simulink model "Copy_of_VTOLTiltrotor"  (R2024a)
settings: configuration reference "VTOLConfiguration" (kept outside this file)
undefined symbols (not defined in the file): airspeed, Battery, BCE12, BCE_Set_init, BMS_Controller_State, C, Cell10_P, Cell11_P, Cell12_P, Cell1_N, Cell1_P, Cell2_P, Cell3_P, Cell4_P, Cell5_P, Cell6_P, Cell7_P, Cell8_P, Cell9_P, Cell_Temperatures, Cell_Voltages, Charging_State, CityMission, control, controlParams, ControlSampleTime, CriticalTiltAngle, currentFactor, CV_Gain, ddx, ddy, ddz, Device_01, DiscIntNeverNeededParam, dx, dy, dz, Earth, env, F, F28379D_ADC_MaxCount, F28379D_ADC_Vmax, FixedWingMission, flightState, Foc_Ki_IxTcpu, Foc_Ki_S, Foc_Kp_I, Foc_Kp_S, fractalcoef, FSState, FWControlParams, HoverMission, I_cc, Ia_offset, Ib_offset, iniRoll, initPitch, iniYaw, IO334, IO334_DAC_Vmax ... (+55)
libraries: slrealtimeethercatlib x109, simulink x81, fl_lib x65, slpidlib x49, mcbcontrolslib x48, nesl_utility x43, speedgoatlib_hdlCoder_IO3xx x31, canmsglib x17, slrealtimeutilitieslib x13, mcbhdlplantlib x13, speedgoatlib_IO611 x12, dspstat3 x12
(part 3 of 20)

== system Copy_of_VTOLTiltrotor/Dynamics/Force and Moments ==
  note: Weather Model - Wind model is disabled by default. To enable wind model, run Wind = 0 and configure the wind model in the Weather Model subsystem.
      |
      | Aerodynamic Forces - Computes aerodynamic forces of the UAV. To modify the aerodynamic derivatives of the UAV, modify the uavParam.aero struct with your own data, or use the Aerodynamic Forces and Moments block from Aerospace Blockset
      |
      | Propulsion - Models the propulsion system. Open this subsystem to configure the rotor direction, tilt angle, etc.
  Actuator : Inport
  CtrlSurfaces : Inport  Port=2
  States : Inport  Port=3
  Add : Sum  Inputs=++++
  Add1 : Sum
  AeroSwitch : Constant  Value=0
  Aerodynamic Drag : Subsystem
  Aerodynamic Forces : Subsystem
  Bus Selector : BusSelector  OutputSignals=DCMbe,Vb
  Bus Selector3 : BusSelector  OutputSignals=Xe,Euler
  Constant4 : Constant  Value=0
  Constant5 : Constant  Value=0
  Gravity : Subsystem
  Propulsion : Subsystem
  Switch : Switch  Criteria=u2 > Threshold  SaturateOnIntegerOverflow=off  InputSameDT=off
  Switch1 : Switch  Criteria=u2 > Threshold  SaturateOnIntegerOverflow=off  InputSameDT=off
  Weather Model : Subsystem  Variant=on  VariantControl=Weather Model
  F : Outport
  M : Outport  Port=2
  RotorParams : Outport  Port=3
  AirData : Outport  Port=4
  wires:
  Bus Selector/1 -> Gravity/1(DCM_be), Aerodynamic Drag/1(DCM_be)  "<DCMbe>"
  Propulsion/3(F) -> Add/1
  Gravity/1(F_g) -> Add/2  "Gravity Force"
  Aerodynamic Drag/1(F_d) -> Add/4  "Drag Force"
  Bus Selector/2 -> Aerodynamic Drag/2(Vb)  "<Vb>"
  Add/1 -> F/1
  States/1 -> Bus Selector3/1, Bus Selector/1, Aerodynamic Forces/4(UAVState), Propulsion/2(States)  "States"
  CtrlSurfaces/1 -> Aerodynamic Forces/3(CtrlSurfaces)
  Add1/1 -> M/1
  Propulsion/2(M) -> Add1/2
  [AeroForce] -> Add/3  "Aerodynamic Force"
  Aerodynamic Forces/2(F) -> Switch/1
  Switch/1 -> [AeroForce]
  Constant4/1 -> Switch/3
  AeroSwitch/1 -> Switch/2, Switch1/2
  Constant5/1 -> Switch1/3
  Switch1/1 -> Add1/1, [AeroMoment]
  Aerodynamic Forces/3(M) -> Switch1/1
  Actuator/1 -> Propulsion/1(Actuator)
  Propulsion/1(RotorParameters) -> RotorParams/1
  Aerodynamic Forces/1(AirData) -> AirData/1, Weather Model/1(AirData)  "Air Data"
  Bus Selector3/1 -> Weather Model/2(Xe)  "<Xe>"
  Bus Selector3/2 -> Weather Model/3(Euler)  "<Euler>"
  Weather Model/1(Wind_e) -> Aerodynamic Forces/1(Wind_e)
  Weather Model/2(Rho) -> Aerodynamic Forces/2(Rho)

== system Copy_of_VTOLTiltrotor/Dynamics/Ground Truth Bus ==
  Ve : Inport
  Xe : Inport  Port=2
  Euler : Inport  Port=3
  DCMbe : Inport  Port=4
  Vb : Inport  Port=5
  pqr : Inport  Port=6
  Abb : Inport  Port=7
  Abe : Inport  Port=8
  RotorParams : Inport  Port=9
  AirData : Inport  Port=10
  Bus Creator : BusCreator  Inputs=13
  Bus Selector : BusSelector  OutputSignals=airspeed
  Direction Cosine Matrix to Quaternions : sharedtransform/Direction Cosine Matrix  to Quaternions  aMode=0  action=None  tolerance=eps(2)
      settings: LibrarySourceBlock=|
      | aerolibtransform2/Direction Cosine Matrix
      | to Quaternions
  MATLAB Function1 : MATLAB Function  TreatAsAtomicUnit=on
  Ground Truth : Outport
  wires:
  pqr/1 -> Bus Creator/6
  Xe/1 -> Bus Creator/2
  Bus Creator/1 -> Ground Truth/1
  DCMbe/1 -> Direction Cosine Matrix to Quaternions/1, Bus Creator/4
  Euler/1 -> Bus Creator/3
  Vb/1 -> Bus Creator/5
  Abb/1 -> Bus Creator/7
  AirData/1 -> Bus Selector/1
  Bus Selector/1 -> Bus Creator/9  "<airspeed>"
  Direction Cosine Matrix to Quaternions/1 -> Bus Creator/10  "q"
  RotorParams/1 -> Bus Creator/8  "RotorParameters"
  Abe/1 -> Bus Creator/11  "Abe"
  MATLAB Function1/2(gndSpeed) -> Bus Creator/13  "gndspeed"
  MATLAB Function1/1(course) -> Bus Creator/12  "course"
  Ve/1 -> MATLAB Function1/1(vxyz), Bus Creator/1

== system Copy_of_VTOLTiltrotor/Dynamics/Variant Subsystem ==
  UAVStates : Inport
  No Sensors : Subsystem  VariantControl=SensorType==0
  Sensors : Subsystem  VariantControl=SensorType==1
  SensorData : Outport

== system Copy_of_VTOLTiltrotor/Flight Controller/Autopilot ==
  note: To modify the output bus interfaces, run open("exampleHelperDefineDigitalTwinInterface.m")
  HoverCommands : Inport
  FixedWingSP : Inport  Port=2
  AAC : Inport  Port=3
  CtrlMode : Inport  Port=4
  FlightMode : Inport  Port=5
  EstimatedStates : Inport  Port=6
  Bus Selector : BusSelector  OutputSignals=inTransition
  Bus Selector1 : BusSelector  OutputSignals=TransitionCondition
  Bus Selector2 : BusSelector  OutputSignals=w1,w2,w3,w4
  Filter or Estimator : Subsystem
  Fixed Wing Controller : Subsystem  Variant=on  VariantControl=Fixed Wing Controller
  Manual Control : Subsystem
  Multicopter Controller : Subsystem
  Scheduler : Subsystem  SystemSampleTime=0.005
  Scope : Scope  NumInputPorts=4
  Tilt Scheduler : Subsystem
  MotorActuatorCommands : Outport
  CtrlSurfaceCmds : Outport  Port=2
  wires:
  EstimatedStates/1 -> Filter or Estimator/1(SensorData)
  Multicopter Controller/1(MixerCommands) -> Scheduler/1(MotorCommands)
  Tilt Scheduler/1(TiltAngle) -> Scheduler/2(TiltSchedule)
  Fixed Wing Controller/1(Actuator) -> Scheduler/6(FixedWingActuators)
  CtrlMode/1 -> Bus Selector1/1, Fixed Wing Controller/2(Control Mode), Bus Selector/1
  Manual Control/1(AERT) -> Fixed Wing Controller/5(AERT)
  Scheduler/1(MotorActuatorCommands) -> Bus Selector2/1, MotorActuatorCommands/1
  Scheduler/2(CtrlSurfaceCommands) -> CtrlSurfaceCmds/1
  HoverCommands/1 -> Multicopter Controller/1(Hover Commands)
  FlightMode/1 -> Tilt Scheduler/1(FlightMode)
  Filter or Estimator/1(States) -> Multicopter Controller/3(States), Fixed Wing Controller/1(States), Tilt Scheduler/2(States), Scheduler/4(States)
  AAC/1 -> Fixed Wing Controller/3(AAC SP)
  FixedWingSP/1 -> Fixed Wing Controller/4(FixedWingSP)
  [TransitionDone] -> Scheduler/5(TransitionDone)
  Tilt Scheduler/2(FlightState) -> Scheduler/3(FlightState)
  Bus Selector/1 -> Multicopter Controller/2(InTransition)  "<inTransition>"
  Bus Selector1/1 -> [TransitionDone]  "<TransitionCondition>"
  Bus Selector2/1 -> Scope/1  "<w1>"
  Bus Selector2/2 -> Scope/2  "<w2>"
  Bus Selector2/3 -> Scope/3  "<w3>"
  Bus Selector2/4 -> Scope/4  "<w4>"

== system Copy_of_VTOLTiltrotor/Flight Controller/Estimator ==
  SensorData : Inport
  Estimation Filter : Subsystem  VariantControl=SensorType==1
  Ground Truth : Subsystem  VariantControl=SensorType==0
  EstimatedStates : Outport

== system Copy_of_VTOLTiltrotor/Flight Controller/Ground Control Station ==
  note: Set mission type. In the project shortcut, choose between:
      | Hover mission by selecting Guidance Mode under Hover
      | Fixed wing mission by selecting Guidance Mode under Fixed wing
      | Transition mission by selecting Set Up Full Transition Mission under Transition
      | City mission by selecting Set Up City Mission under Photorealistic Simulation
  UAVState : Inport
  Get Flight Mission : Subsystem  Variant=on  VariantControlMode=label  LabelModeActiveChoice=useQGC==0
  Global Mission : Outport
  wires:
  Get Flight Mission/1("Mission ") -> Global Mission/1
  UAVState/1 -> Get Flight Mission/1(UAVState)

== system Copy_of_VTOLTiltrotor/Flight Controller/Guidance Test Bench ==
  note: Set control type. In the project shortcut, choose between:
      | 1. Manual control by selecting Manual Mode under Hover and open the subsystem to manually control the UAV in hover mode.
      | 2. Guidance testbench with prebuilt mission by selecting Guidance Mod e in the project shortcut.
  Aircraft States : Inport
  Global Mission : Inport  Port=2
  ControlType : Subsystem  Variant=on  VariantControl=Choice
  Rate Transition : RateTransition  OutPortSampleTime=0.005
  "Reference Tracking " : Subsystem
      settings: PortSchema="{\"entries\":[{\"content\":{\"sides\":[{\"content\":{\"connectorIds\":[\"In1\"]},\"type\":\"ConnectorPlacement.EquallySpacedRectSide\",\"uuid\":\"259d5f1e-a362-4dc0-8429-ef92dd781b31\"},{\"content\":{\"connectorIds\":[\"In2\",\"In3\"],\"side\":\"RIGHT\"},\"type\":\"ConnectorPlacement.EquallySpacedRectSide\",\"uuid\":\"8f699bfb-ab92-4bfa-94de-3c6c350a8a94\"},{\"content\":{\"connectorIds\":[],\"side\":\"TOP\"},\"type\":\"ConnectorPlacement.EquallySpacedRectSide\",\"uuid\":\"95dbffc6-e5b7-446a-adcb-afa0cff8c552\"}]},\"type\":\"ConnectorPlacement.EquallySpacedConnector\",\"uuid\":\"e657b5d9-4fa5-41f8-85e3-18a1074ff1cd\"}],\"packageUris\":[\"http://schema.mathworks.com/mf0/Connector/R2020b\"],\"version\":\"1.0\"}"
  HoverSP : Outport
  FixedWingSP : Outport  Port=2
  AACSP : Outport  Port=3
  ctrlMode : Outport  Port=4
  FlightMode : Outport  Port=5
  wires:
  Aircraft States/1 -> Rate Transition/1
  ControlType/1(HoverCmds) -> "Reference Tracking "/2(Position Command), HoverSP/1
  Global Mission/1 -> ControlType/2(Global Mission)
  ControlType/2(FixedWingSP) -> FixedWingSP/1
  ControlType/5(FlightMode) -> FlightMode/1
  ControlType/4(ctrlMode) -> ctrlMode/1
  ControlType/3(AACSP) -> "Reference Tracking "/3(AAC Commands), AACSP/1
  Rate Transition/1 -> "Reference Tracking "/1(State), ControlType/1(Aircraft States)

== system Copy_of_VTOLTiltrotor/Motor Control/Actuator To PWM for all motors ==
  Motor Commands : Inport
  Bus Creator : BusCreator  Inputs=6  OutDataTypeStr=Bus: RotorCntrlBus
  Bus Selector : BusSelector  OutputSignals=w1,w2,w3,w4,Tilt1,Tilt2
  Gain{,1..2,4} (4 alike) : Gain  Gain=1/(uavParam.motor.RPMMAX/60)
  Gain3 : Gain  Gain=1/(pi/2)
  Gain5 : Gain  Gain=1/(pi/2)
  To PWM : Outport
  wires:
  Motor Commands/1 -> Bus Selector/1
  Bus Selector/1 -> Gain/1  "<w1>"
  Bus Selector/3 -> Gain1/1  "<w3>"
  Bus Selector/2 -> Gain4/1  "<w2>"
  Bus Selector/4 -> Gain2/1  "<w4>"
  Bus Selector/5 -> Gain3/1  "<Tilt1>"
  Bus Selector/6 -> Gain5/1  "<Tilt2>"
  Gain/1 -> Bus Creator/1  "w1"
  Gain4/1 -> Bus Creator/2  "w2"
  Gain1/1 -> Bus Creator/3  "w3"
  Gain2/1 -> Bus Creator/4  "w4"
  Gain3/1 -> Bus Creator/5  "Tilt1"
  Gain5/1 -> Bus Creator/6  "Tilt2"
  Bus Creator/1 -> To PWM/1

== system Copy_of_VTOLTiltrotor/Motor Control/Actuator To RPM for 1 motor ==
  Motor Commands : Inport
  Gain : Gain  Gain=10
  Selector : Selector  InputPortWidth=6  IndexOptions=Index vector (dialog)  Indices=[1]  OutputSizes=1
  RPM : Outport
  wires:
  Motor Commands/1 -> Selector/1
  Selector/1 -> Gain/1
  Gain/1 -> RPM/1

== system Copy_of_VTOLTiltrotor/Motor Control/Actuator To RPM for 1 motor1 ==
  Motor Commands : Inport
  Gain : Gain  Gain=10
  Selector : Selector  InputPortWidth=6  IndexOptions=Index vector (dialog)  Indices=[2]  OutputSizes=1
  RPM : Outport
  wires:
  Motor Commands/1 -> Selector/1
  Selector/1 -> Gain/1
  Gain/1 -> RPM/1

== system Copy_of_VTOLTiltrotor/Motor Control/Actuator To RPM for 1 motor2 ==
  Motor Commands : Inport
  Gain : Gain  Gain=10
  Selector : Selector  InputPortWidth=6  IndexOptions=Index vector (dialog)  Indices=[3]  OutputSizes=1
  RPM : Outport
  wires:
  Motor Commands/1 -> Selector/1
  Selector/1 -> Gain/1
  Gain/1 -> RPM/1

== system Copy_of_VTOLTiltrotor/Motor Control/Actuator To RPM for 1 motor3 ==
  Motor Commands : Inport
  Gain : Gain  Gain=10
  Selector : Selector  InputPortWidth=6  IndexOptions=Index vector (dialog)  Indices=[4]  OutputSizes=1
  RPM : Outport
  wires:
  Motor Commands/1 -> Selector/1
  Selector/1 -> Gain/1
  Gain/1 -> RPM/1

== system Copy_of_VTOLTiltrotor/Motor Control/Controller ==
  Iab : Inport
  QAE_MIL_fbk : Inport  Port=2
  EnablePWM : Inport  Port=3
  Closed_Loop_FOC : Inport  Port=4
  Speed_CMD_RPM : Inport  Port=5
  Controller_Parameters : Inport  Port=6
  Controller_HIL_CAN : Subsystem  VariantControl=strcmp(get_param(['VTOLTiltrotor/Motor Control/SimulationVariant'], 'Value'),'3')
  Controller_MIL : Subsystem  VariantControl=(default)
  Controller_fbk : Outport
  Simu_config : Outport  Port=2

== system Copy_of_VTOLTiltrotor/Motor Control/Controller Parameters ==
  Controller_Parameters : BusCreator  Inputs=6
  Controller_Parameters1 : BusCreator  Inputs=6
  Default Values : Constant  OutDataTypeStr=boolean  SampleTime=Ts_UI
  Foc_Ki_S : Constant  Value=Foc_Ki_S  OutDataTypeStr=single
  Foc_Kp_I : Constant  Value=Foc_Kp_I  OutDataTypeStr=single
  Foc_Kp_S : Constant  Value=Foc_Kp_S  OutDataTypeStr=single
  Ia Offset : Constant  Value=Ia_offset  OutDataTypeStr=single
  Ia_offset : Constant  Value=Ia_offset  OutDataTypeStr=single  SampleTime=Ts_UI
  Ib Offset : Constant  Value=Ib_offset  OutDataTypeStr=single
  Ib_offset : Constant  Value=Ib_offset  OutDataTypeStr=single  SampleTime=Ts_UI
  Ki_S : Constant  Value=0.1  OutDataTypeStr=single  SampleTime=Ts_UI
  Ki_i*Tcpu : Constant  Value=Foc_Ki_IxTcpu  OutDataTypeStr=single  SampleTime=Ts_UI
  Ki_i*Tcpu1 : Constant  Value=Foc_Ki_IxTcpu  OutDataTypeStr=single
  Kp_I : Constant  Value=Foc_Kp_I  OutDataTypeStr=single  SampleTime=Ts_UI
  Kp_S : Constant  Value=0.1  OutDataTypeStr=single  SampleTime=Ts_UI
  Rate Transition : RateTransition  OutPortSampleTime=Ts_UI
  Switch : Switch  Criteria=u2 ~= 0  SaturateOnIntegerOverflow=off  InputSameDT=off
  Controller Parameters : Outport
  wires:
  Ia_offset/1 -> Controller_Parameters/5  "Ia_offset"
  Foc_Kp_S/1 -> Controller_Parameters1/1  "Kp_S"
  Ia Offset/1 -> Controller_Parameters1/5  "Ia_offset"
  Ib Offset/1 -> Controller_Parameters1/6  "Ib_offset"
  Controller_Parameters/1 -> Switch/3
  Foc_Ki_S/1 -> Controller_Parameters1/2  "Ki_S"
  Foc_Kp_I/1 -> Controller_Parameters1/3  "Kp_I"
  Controller_Parameters1/1 -> Rate Transition/1
  Ib_offset/1 -> Controller_Parameters/6  "Ib_offset"
  Ki_i*Tcpu/1 -> Controller_Parameters/4  "Ki_IxTcpu"
  Ki_S/1 -> Controller_Parameters/2  "Ki_S"
  Ki_i*Tcpu1/1 -> Controller_Parameters1/4  "Ki_IxTcpu"
  Kp_I/1 -> Controller_Parameters/3  "Kp_I"
  Kp_S/1 -> Controller_Parameters/1  "Kp_S"
  Switch/1 -> Controller Parameters/1
  Rate Transition/1 -> Switch/1
  Default Values/1 -> Switch/2  "Default Values"

== system Copy_of_VTOLTiltrotor/Motor Control/Controller Parameters1 ==
  Controller_Parameters : BusCreator  Inputs=6
  Controller_Parameters1 : BusCreator  Inputs=6
  Default Values : Constant  OutDataTypeStr=boolean  SampleTime=Ts_UI
  Foc_Ki_S : Constant  Value=Foc_Ki_S  OutDataTypeStr=single
  Foc_Kp_I : Constant  Value=Foc_Kp_I  OutDataTypeStr=single
  Foc_Kp_S : Constant  Value=Foc_Kp_S  OutDataTypeStr=single
  Ia Offset : Constant  Value=Ia_offset  OutDataTypeStr=single
  Ia_offset : Constant  Value=Ia_offset  OutDataTypeStr=single  SampleTime=Ts_UI
  Ib Offset : Constant  Value=Ib_offset  OutDataTypeStr=single
  Ib_offset : Constant  Value=Ib_offset  OutDataTypeStr=single  SampleTime=Ts_UI
  Ki_S : Constant  Value=0.1  OutDataTypeStr=single  SampleTime=Ts_UI
  Ki_i*Tcpu : Constant  Value=Foc_Ki_IxTcpu  OutDataTypeStr=single  SampleTime=Ts_UI
  Ki_i*Tcpu1 : Constant  Value=Foc_Ki_IxTcpu  OutDataTypeStr=single
  Kp_I : Constant  Value=Foc_Kp_I  OutDataTypeStr=single  SampleTime=Ts_UI
  Kp_S : Constant  Value=0.1  OutDataTypeStr=single  SampleTime=Ts_UI
  Rate Transition : RateTransition  OutPortSampleTime=Ts_UI
  Switch : Switch  Criteria=u2 ~= 0  SaturateOnIntegerOverflow=off  InputSameDT=off
  Controller Parameters : Outport
  wires:
  Ia_offset/1 -> Controller_Parameters/5  "Ia_offset"
  Foc_Kp_S/1 -> Controller_Parameters1/1  "Kp_S"
  Ia Offset/1 -> Controller_Parameters1/5  "Ia_offset"
  Ib Offset/1 -> Controller_Parameters1/6  "Ib_offset"
  Controller_Parameters/1 -> Switch/3
  Foc_Ki_S/1 -> Controller_Parameters1/2  "Ki_S"
  Foc_Kp_I/1 -> Controller_Parameters1/3  "Kp_I"
  Controller_Parameters1/1 -> Rate Transition/1
  Ib_offset/1 -> Controller_Parameters/6  "Ib_offset"
  Ki_i*Tcpu/1 -> Controller_Parameters/4  "Ki_IxTcpu"
  Ki_S/1 -> Controller_Parameters/2  "Ki_S"
  Ki_i*Tcpu1/1 -> Controller_Parameters1/4  "Ki_IxTcpu"
  Kp_I/1 -> Controller_Parameters/3  "Kp_I"
  Kp_S/1 -> Controller_Parameters/1  "Kp_S"
  Switch/1 -> Controller Parameters/1
  Rate Transition/1 -> Switch/1
  Default Values/1 -> Switch/2  "Default Values"

== system Copy_of_VTOLTiltrotor/Motor Control/Controller Parameters2 ==
  Controller_Parameters : BusCreator  Inputs=6
  Controller_Parameters1 : BusCreator  Inputs=6
  Default Values : Constant  OutDataTypeStr=boolean  SampleTime=Ts_UI
  Foc_Ki_S : Constant  Value=Foc_Ki_S  OutDataTypeStr=single
  Foc_Kp_I : Constant  Value=Foc_Kp_I  OutDataTypeStr=single
  Foc_Kp_S : Constant  Value=Foc_Kp_S  OutDataTypeStr=single
  Ia Offset : Constant  Value=Ia_offset  OutDataTypeStr=single
  Ia_offset : Constant  Value=Ia_offset  OutDataTypeStr=single  SampleTime=Ts_UI
  Ib Offset : Constant  Value=Ib_offset  OutDataTypeStr=single
  Ib_offset : Constant  Value=Ib_offset  OutDataTypeStr=single  SampleTime=Ts_UI
  Ki_S : Constant  Value=0.1  OutDataTypeStr=single  SampleTime=Ts_UI
  Ki_i*Tcpu : Constant  Value=Foc_Ki_IxTcpu  OutDataTypeStr=single  SampleTime=Ts_UI
  Ki_i*Tcpu1 : Constant  Value=Foc_Ki_IxTcpu  OutDataTypeStr=single
  Kp_I : Constant  Value=Foc_Kp_I  OutDataTypeStr=single  SampleTime=Ts_UI
  Kp_S : Constant  Value=0.1  OutDataTypeStr=single  SampleTime=Ts_UI
  Rate Transition : RateTransition  OutPortSampleTime=Ts_UI
  Switch : Switch  Criteria=u2 ~= 0  SaturateOnIntegerOverflow=off  InputSameDT=off
  Controller Parameters : Outport
  wires:
  Ia_offset/1 -> Controller_Parameters/5  "Ia_offset"
  Foc_Kp_S/1 -> Controller_Parameters1/1  "Kp_S"
  Ia Offset/1 -> Controller_Parameters1/5  "Ia_offset"
  Ib Offset/1 -> Controller_Parameters1/6  "Ib_offset"
  Controller_Parameters/1 -> Switch/3
  Foc_Ki_S/1 -> Controller_Parameters1/2  "Ki_S"
  Foc_Kp_I/1 -> Controller_Parameters1/3  "Kp_I"
  Controller_Parameters1/1 -> Rate Transition/1
  Ib_offset/1 -> Controller_Parameters/6  "Ib_offset"
  Ki_i*Tcpu/1 -> Controller_Parameters/4  "Ki_IxTcpu"
  Ki_S/1 -> Controller_Parameters/2  "Ki_S"
  Ki_i*Tcpu1/1 -> Controller_Parameters1/4  "Ki_IxTcpu"
  Kp_I/1 -> Controller_Parameters/3  "Kp_I"
  Kp_S/1 -> Controller_Parameters/1  "Kp_S"
  Switch/1 -> Controller Parameters/1
  Rate Transition/1 -> Switch/1
  Default Values/1 -> Switch/2  "Default Values"

== system Copy_of_VTOLTiltrotor/Motor Control/Controller Parameters3 ==
  Controller_Parameters : BusCreator  Inputs=6
  Controller_Parameters1 : BusCreator  Inputs=6
  Default Values : Constant  OutDataTypeStr=boolean  SampleTime=Ts_UI
  Foc_Ki_S : Constant  Value=Foc_Ki_S  OutDataTypeStr=single
  Foc_Kp_I : Constant  Value=Foc_Kp_I  OutDataTypeStr=single
  Foc_Kp_S : Constant  Value=Foc_Kp_S  OutDataTypeStr=single
  Ia Offset : Constant  Value=Ia_offset  OutDataTypeStr=single
  Ia_offset : Constant  Value=Ia_offset  OutDataTypeStr=single  SampleTime=Ts_UI
  Ib Offset : Constant  Value=Ib_offset  OutDataTypeStr=single
  Ib_offset : Constant  Value=Ib_offset  OutDataTypeStr=single  SampleTime=Ts_UI
  Ki_S : Constant  Value=0.1  OutDataTypeStr=single  SampleTime=Ts_UI
  Ki_i*Tcpu : Constant  Value=Foc_Ki_IxTcpu  OutDataTypeStr=single  SampleTime=Ts_UI
  Ki_i*Tcpu1 : Constant  Value=Foc_Ki_IxTcpu  OutDataTypeStr=single
  Kp_I : Constant  Value=Foc_Kp_I  OutDataTypeStr=single  SampleTime=Ts_UI
  Kp_S : Constant  Value=0.1  OutDataTypeStr=single  SampleTime=Ts_UI
  Rate Transition : RateTransition  OutPortSampleTime=Ts_UI
  Switch : Switch  Criteria=u2 ~= 0  SaturateOnIntegerOverflow=off  InputSameDT=off
  Controller Parameters : Outport
  wires:
  Ia_offset/1 -> Controller_Parameters/5  "Ia_offset"
  Foc_Kp_S/1 -> Controller_Parameters1/1  "Kp_S"
  Ia Offset/1 -> Controller_Parameters1/5  "Ia_offset"
  Ib Offset/1 -> Controller_Parameters1/6  "Ib_offset"
  Controller_Parameters/1 -> Switch/3
  Foc_Ki_S/1 -> Controller_Parameters1/2  "Ki_S"
  Foc_Kp_I/1 -> Controller_Parameters1/3  "Kp_I"
  Controller_Parameters1/1 -> Rate Transition/1
  Ib_offset/1 -> Controller_Parameters/6  "Ib_offset"
  Ki_i*Tcpu/1 -> Controller_Parameters/4  "Ki_IxTcpu"
  Ki_S/1 -> Controller_Parameters/2  "Ki_S"
  Ki_i*Tcpu1/1 -> Controller_Parameters1/4  "Ki_IxTcpu"
  Kp_I/1 -> Controller_Parameters/3  "Kp_I"
  Kp_S/1 -> Controller_Parameters/1  "Kp_S"
  Switch/1 -> Controller Parameters/1
  Rate Transition/1 -> Switch/1
  Default Values/1 -> Switch/2  "Default Values"

== system Copy_of_VTOLTiltrotor/Motor Control/Controller1 ==
  Iab : Inport
  QAE_MIL_fbk : Inport  Port=2
  EnablePWM : Inport  Port=3
  Closed_Loop_FOC : Inport  Port=4
  Speed_CMD_RPM : Inport  Port=5
  Controller_Parameters : Inport  Port=6
  Controller_MIL : Subsystem  VariantControl=(default)
  Controller_fbk : Outport
  Simu_config : Outport  Port=2

== system Copy_of_VTOLTiltrotor/Motor Control/Controller2 ==
  Iab : Inport
  QAE_MIL_fbk : Inport  Port=2
  EnablePWM : Inport  Port=3
  Closed_Loop_FOC : Inport  Port=4
  Speed_CMD_RPM : Inport  Port=5
  Controller_Parameters : Inport  Port=6
  Controller_MIL : Subsystem  VariantControl=(default)
  Controller_fbk : Outport
  Simu_config : Outport  Port=2

== system Copy_of_VTOLTiltrotor/Motor Control/Controller3 ==
  Iab : Inport
  QAE_MIL_fbk : Inport  Port=2
  EnablePWM : Inport  Port=3
  Closed_Loop_FOC : Inport  Port=4
  Speed_CMD_RPM : Inport  Port=5
  Controller_Parameters : Inport  Port=6
  Controller_MIL : Subsystem  VariantControl=(default)
  Controller_fbk : Outport
  Simu_config : Outport  Port=2

== system Copy_of_VTOLTiltrotor/Motor Control/Controller_fbk_signals ==
  Controller_fbk : Inport
  Data Type Conversion : DataTypeConversion  OutDataTypeStr=boolean  SaturateOnIntegerOverflow=off  RndMeth=Floor
  Demux : Demux
  Terminator{,1..3} (4 alike) : Terminator
  wires:
  Demux/1 -> Terminator1/1  "Speed_fbk"
  Controller_fbk/1 -> Demux/1
  Demux/2 -> Terminator3/1  "Encoder_Pos_fbk"
  Demux/4 -> Data Type Conversion/1  "Spd_Pot_fdk"
  Demux/3 -> Terminator2/1  "Speed_Cmd_fbk"
  Data Type Conversion/1 -> Terminator/1  "Spd_pot_enable"

== system Copy_of_VTOLTiltrotor/Motor Control/Controller_fbk_signals1 ==
  Controller_fbk : Inport
  Data Type Conversion : DataTypeConversion  OutDataTypeStr=boolean  SaturateOnIntegerOverflow=off  RndMeth=Floor
  Demux : Demux
  Terminator{,1..3} (4 alike) : Terminator
  wires:
  Demux/1 -> Terminator1/1  "Speed_fbk"
  Controller_fbk/1 -> Demux/1
  Demux/2 -> Terminator3/1  "Encoder_Pos_fbk"
  Demux/4 -> Data Type Conversion/1  "Spd_Pot_fdk"
  Demux/3 -> Terminator2/1  "Speed_Cmd_fbk"
  Data Type Conversion/1 -> Terminator/1  "Spd_pot_enable"

== system Copy_of_VTOLTiltrotor/Motor Control/Controller_fbk_signals2 ==
  Controller_fbk : Inport
  Data Type Conversion : DataTypeConversion  OutDataTypeStr=boolean  SaturateOnIntegerOverflow=off  RndMeth=Floor
  Demux : Demux
  Terminator{,1..3} (4 alike) : Terminator
  wires:
  Demux/1 -> Terminator1/1  "Speed_fbk"
  Controller_fbk/1 -> Demux/1
  Demux/2 -> Terminator3/1  "Encoder_Pos_fbk"
  Demux/4 -> Data Type Conversion/1  "Spd_Pot_fdk"
  Demux/3 -> Terminator2/1  "Speed_Cmd_fbk"
  Data Type Conversion/1 -> Terminator/1  "Spd_pot_enable"

== system Copy_of_VTOLTiltrotor/Motor Control/Controller_fbk_signals3 ==
  Controller_fbk : Inport
  Data Type Conversion : DataTypeConversion  OutDataTypeStr=boolean  SaturateOnIntegerOverflow=off  RndMeth=Floor
  Demux : Demux
  Terminator{,1..3} (4 alike) : Terminator
  wires:
  Demux/1 -> Terminator1/1  "Speed_fbk"
  Controller_fbk/1 -> Demux/1
  Demux/2 -> Terminator3/1  "Encoder_Pos_fbk"
  Demux/4 -> Data Type Conversion/1  "Spd_Pot_fdk"
  Demux/3 -> Terminator2/1  "Speed_Cmd_fbk"
  Data Type Conversion/1 -> Terminator/1  "Spd_pot_enable"

== system Copy_of_VTOLTiltrotor/Motor Control/Fault Trigering ==
  AND : Logic  Inputs=3  IconShape=distinctive  AllPortsSameDT=off  OutDataTypeStr=boolean
  Bit to Integer Converter : simulink/Logic and Bit Operations/Bit to Integer Converter  nbits=32  bitOrder=LSB first  signedOutputValues=Unsigned  outDtype=uint32  outDtypeSigned=Inherit via internal rule
  Close_An : Constant  Value=0  OutDataTypeStr=boolean  SampleTime=Ts_UI
  Close_Ap : Constant  Value=0  OutDataTypeStr=boolean  SampleTime=Ts_UI
  Close_Bn : Constant  Value=0  OutDataTypeStr=boolean  SampleTime=Ts_UI
  Close_Bp : Constant  Value=0  OutDataTypeStr=boolean  SampleTime=Ts_UI
  Close_Cn : Constant  Value=0  OutDataTypeStr=boolean  SampleTime=Ts_UI
  Close_Cp : Constant  Value=0  OutDataTypeStr=boolean  SampleTime=Ts_UI
  Constant1 : Constant  Value=0  OutDataTypeStr=uint32
  Constant{14..15,20..25,32..36} (13 alike) : Constant  Value=0  OutDataTypeStr=boolean  SampleTime=Ts_UI
  Constant2 : Constant  OutDataTypeStr=boolean  SampleTime=Ts_UI
  Enable_Fault_UI : Constant  OutDataTypeStr=boolean  SampleTime=Ts_UI
  OR : Logic  Operator=OR  Inputs=18  IconShape=distinctive  AllPortsSameDT=off  OutDataTypeStr=boolean
  Open_An : Constant  Value=0  OutDataTypeStr=boolean  SampleTime=Ts_UI
  Open_Ap : Constant  Value=0  OutDataTypeStr=boolean  SampleTime=Ts_UI
  Open_Bn : Constant  Value=0  OutDataTypeStr=boolean  SampleTime=Ts_UI
  Open_Bp : Constant  Value=0  OutDataTypeStr=boolean  SampleTime=Ts_UI
  Open_Cn : Constant  Value=0  OutDataTypeStr=boolean  SampleTime=Ts_UI
  Open_Cp : Constant  Value=0  OutDataTypeStr=boolean  SampleTime=Ts_UI
  Short_A : Constant  Value=0  OutDataTypeStr=boolean  SampleTime=Ts_UI
  Short_AB : Constant  Value=0  OutDataTypeStr=boolean  SampleTime=Ts_UI
  Short_B : Constant  Value=0  OutDataTypeStr=boolean  SampleTime=Ts_UI
  Short_BC : Constant  Value=0  OutDataTypeStr=boolean  SampleTime=Ts_UI
  Short_C : Constant  Value=0  OutDataTypeStr=boolean  SampleTime=Ts_UI
  Short_CA : Constant  Value=0  OutDataTypeStr=boolean  SampleTime=Ts_UI
  Switch : Switch  Criteria=u2 > Threshold  SaturateOnIntegerOverflow=off  InputSameDT=off
  Terminator : Terminator
  Vector Concatenate : Concatenate  NumInputs=32
  Faults : Outport
  wires:
  Open_Cn/1 -> OR/12, Vector Concatenate/12
  Open_Cp/1 -> OR/9, Vector Concatenate/9
  Short_A/1 -> OR/1, Vector Concatenate/1
  Open_Bp/1 -> OR/8, Vector Concatenate/8
  Short_B/1 -> Vector Concatenate/2, OR/2
  Short_C/1 -> Vector Concatenate/3, OR/3
  Short_AB/1 -> Vector Concatenate/4, OR/4
  Short_BC/1 -> Vector Concatenate/5, OR/5
  Short_CA/1 -> OR/6, Vector Concatenate/6
  Constant36/1 -> Vector Concatenate/31
  Open_Bn/1 -> OR/11, Vector Concatenate/11
  Open_An/1 -> OR/10, Vector Concatenate/10
  Open_Ap/1 -> OR/7, Vector Concatenate/7
  Close_An/1 -> OR/16, Vector Concatenate/16
  Close_Ap/1 -> OR/13, Vector Concatenate/13
  Close_Cn/1 -> OR/18, Vector Concatenate/18
  Close_Bn/1 -> OR/17, Vector Concatenate/17
  Close_Cp/1 -> OR/15, Vector Concatenate/15
  Close_Bp/1 -> OR/14, Vector Concatenate/14
  Constant15/1 -> Vector Concatenate/24
  Constant14/1 -> Vector Concatenate/23
  Constant21/1 -> Vector Concatenate/20
  Constant20/1 -> Vector Concatenate/19
  Constant25/1 -> Vector Concatenate/26
  Constant24/1 -> Vector Concatenate/25
  Constant23/1 -> Vector Concatenate/22
  Constant22/1 -> Vector Concatenate/21
  Constant35/1 -> Vector Concatenate/30
  Constant34/1 -> Vector Concatenate/29
  Constant33/1 -> Vector Concatenate/28
  Constant32/1 -> Vector Concatenate/27
  Enable_Fault_UI/1 -> AND/3, Switch/2
  Vector Concatenate/1 -> Bit to Integer Converter/1
  Switch/1 -> Faults/1
  Bit to Integer Converter/1 -> Switch/1
  Constant1/1 -> Switch/3
  OR/1 -> AND/1
  AND/1 -> Terminator/1  "Fault_Present"
  Constant2/1 -> AND/2, Vector Concatenate/32

== system Copy_of_VTOLTiltrotor/Motor Control/Fault Trigering1 ==
  AND : Logic  Inputs=3  IconShape=distinctive  AllPortsSameDT=off  OutDataTypeStr=boolean
  Bit to Integer Converter : simulink/Logic and Bit Operations/Bit to Integer Converter  nbits=32  bitOrder=LSB first  signedOutputValues=Unsigned  outDtype=uint32  outDtypeSigned=Inherit via internal rule
  Close_An : Constant  Value=0  OutDataTypeStr=boolean  SampleTime=Ts_UI
  Close_Ap : Constant  Value=0  OutDataTypeStr=boolean  SampleTime=Ts_UI
  Close_Bn : Constant  Value=0  OutDataTypeStr=boolean  SampleTime=Ts_UI
  Close_Bp : Constant  Value=0  OutDataTypeStr=boolean  SampleTime=Ts_UI
  Close_Cn : Constant  Value=0  OutDataTypeStr=boolean  SampleTime=Ts_UI
  Close_Cp : Constant  Value=0  OutDataTypeStr=boolean  SampleTime=Ts_UI
  Constant1 : Constant  Value=0  OutDataTypeStr=uint32
  Constant{14..15,20..25,32..36} (13 alike) : Constant  Value=0  OutDataTypeStr=boolean  SampleTime=Ts_UI
  Constant2 : Constant  OutDataTypeStr=boolean  SampleTime=Ts_UI
  Enable_Fault_UI : Constant  OutDataTypeStr=boolean  SampleTime=Ts_UI
  OR : Logic  Operator=OR  Inputs=18  IconShape=distinctive  AllPortsSameDT=off  OutDataTypeStr=boolean
  Open_An : Constant  Value=0  OutDataTypeStr=boolean  SampleTime=Ts_UI
  Open_Ap : Constant  Value=0  OutDataTypeStr=boolean  SampleTime=Ts_UI
  Open_Bn : Constant  Value=0  OutDataTypeStr=boolean  SampleTime=Ts_UI
  Open_Bp : Constant  Value=0  OutDataTypeStr=boolean  SampleTime=Ts_UI
  Open_Cn : Constant  Value=0  OutDataTypeStr=boolean  SampleTime=Ts_UI
  Open_Cp : Constant  Value=0  OutDataTypeStr=boolean  SampleTime=Ts_UI
  Short_A : Constant  Value=0  OutDataTypeStr=boolean  SampleTime=Ts_UI
  Short_AB : Constant  Value=0  OutDataTypeStr=boolean  SampleTime=Ts_UI
  Short_B : Constant  Value=0  OutDataTypeStr=boolean  SampleTime=Ts_UI
  Short_BC : Constant  Value=0  OutDataTypeStr=boolean  SampleTime=Ts_UI
  Short_C : Constant  Value=0  OutDataTypeStr=boolean  SampleTime=Ts_UI
  Short_CA : Constant  Value=0  OutDataTypeStr=boolean  SampleTime=Ts_UI
  Switch : Switch  Criteria=u2 > Threshold  SaturateOnIntegerOverflow=off  InputSameDT=off
  Terminator : Terminator
  Vector Concatenate : Concatenate  NumInputs=32
  Faults : Outport
  wires:
  Open_Cn/1 -> OR/12, Vector Concatenate/12
  Open_Cp/1 -> OR/9, Vector Concatenate/9
  Short_A/1 -> OR/1, Vector Concatenate/1
  Open_Bp/1 -> OR/8, Vector Concatenate/8
  Short_B/1 -> Vector Concatenate/2, OR/2
  Short_C/1 -> Vector Concatenate/3, OR/3
  Short_AB/1 -> Vector Concatenate/4, OR/4
  Short_BC/1 -> Vector Concatenate/5, OR/5
  Short_CA/1 -> OR/6, Vector Concatenate/6
  Constant36/1 -> Vector Concatenate/31
  Open_Bn/1 -> OR/11, Vector Concatenate/11
  Open_An/1 -> OR/10, Vector Concatenate/10
  Open_Ap/1 -> OR/7, Vector Concatenate/7
  Close_An/1 -> OR/16, Vector Concatenate/16
  Close_Ap/1 -> OR/13, Vector Concatenate/13
  Close_Cn/1 -> OR/18, Vector Concatenate/18
  Close_Bn/1 -> OR/17, Vector Concatenate/17
  Close_Cp/1 -> OR/15, Vector Concatenate/15
  Close_Bp/1 -> OR/14, Vector Concatenate/14
  Constant15/1 -> Vector Concatenate/24
  Constant14/1 -> Vector Concatenate/23
  Constant21/1 -> Vector Concatenate/20
  Constant20/1 -> Vector Concatenate/19
  Constant25/1 -> Vector Concatenate/26
  Constant24/1 -> Vector Concatenate/25
  Constant23/1 -> Vector Concatenate/22
  Constant22/1 -> Vector Concatenate/21
  Constant35/1 -> Vector Concatenate/30
  Constant34/1 -> Vector Concatenate/29
  Constant33/1 -> Vector Concatenate/28
  Constant32/1 -> Vector Concatenate/27
  Enable_Fault_UI/1 -> AND/3, Switch/2
  Vector Concatenate/1 -> Bit to Integer Converter/1
  Switch/1 -> Faults/1
  Bit to Integer Converter/1 -> Switch/1
  Constant1/1 -> Switch/3
  OR/1 -> AND/1
  AND/1 -> Terminator/1  "Fault_Present"
  Constant2/1 -> AND/2, Vector Concatenate/32

== system Copy_of_VTOLTiltrotor/Motor Control/Fault Trigering2 ==
  AND : Logic  Inputs=3  IconShape=distinctive  AllPortsSameDT=off  OutDataTypeStr=boolean
  Bit to Integer Converter : simulink/Logic and Bit Operations/Bit to Integer Converter  nbits=32  bitOrder=LSB first  signedOutputValues=Unsigned  outDtype=uint32  outDtypeSigned=Inherit via internal rule
  Close_An : Constant  Value=0  OutDataTypeStr=boolean  SampleTime=Ts_UI
  Close_Ap : Constant  Value=0  OutDataTypeStr=boolean  SampleTime=Ts_UI
  Close_Bn : Constant  Value=0  OutDataTypeStr=boolean  SampleTime=Ts_UI
  Close_Bp : Constant  Value=0  OutDataTypeStr=boolean  SampleTime=Ts_UI
  Close_Cn : Constant  Value=0  OutDataTypeStr=boolean  SampleTime=Ts_UI
  Close_Cp : Constant  Value=0  OutDataTypeStr=boolean  SampleTime=Ts_UI
  Constant1 : Constant  Value=0  OutDataTypeStr=uint32
  Constant{14..15,20..25,32..36} (13 alike) : Constant  Value=0  OutDataTypeStr=boolean  SampleTime=Ts_UI
  Constant2 : Constant  OutDataTypeStr=boolean  SampleTime=Ts_UI
  Enable_Fault_UI : Constant  OutDataTypeStr=boolean  SampleTime=Ts_UI
  OR : Logic  Operator=OR  Inputs=18  IconShape=distinctive  AllPortsSameDT=off  OutDataTypeStr=boolean
  Open_An : Constant  Value=0  OutDataTypeStr=boolean  SampleTime=Ts_UI
  Open_Ap : Constant  Value=0  OutDataTypeStr=boolean  SampleTime=Ts_UI
  Open_Bn : Constant  Value=0  OutDataTypeStr=boolean  SampleTime=Ts_UI
  Open_Bp : Constant  Value=0  OutDataTypeStr=boolean  SampleTime=Ts_UI
  Open_Cn : Constant  Value=0  OutDataTypeStr=boolean  SampleTime=Ts_UI
  Open_Cp : Constant  Value=0  OutDataTypeStr=boolean  SampleTime=Ts_UI
  Short_A : Constant  Value=0  OutDataTypeStr=boolean  SampleTime=Ts_UI
  Short_AB : Constant  Value=0  OutDataTypeStr=boolean  SampleTime=Ts_UI
  Short_B : Constant  Value=0  OutDataTypeStr=boolean  SampleTime=Ts_UI
  Short_BC : Constant  Value=0  OutDataTypeStr=boolean  SampleTime=Ts_UI
  Short_C : Constant  Value=0  OutDataTypeStr=boolean  SampleTime=Ts_UI
  Short_CA : Constant  Value=0  OutDataTypeStr=boolean  SampleTime=Ts_UI
  Switch : Switch  Criteria=u2 > Threshold  SaturateOnIntegerOverflow=off  InputSameDT=off
  Terminator : Terminator
  Vector Concatenate : Concatenate  NumInputs=32
  Faults : Outport
  wires:
  Open_Cn/1 -> OR/12, Vector Concatenate/12
  Open_Cp/1 -> OR/9, Vector Concatenate/9
  Short_A/1 -> OR/1, Vector Concatenate/1
  Open_Bp/1 -> OR/8, Vector Concatenate/8
  Short_B/1 -> Vector Concatenate/2, OR/2
  Short_C/1 -> Vector Concatenate/3, OR/3
  Short_AB/1 -> Vector Concatenate/4, OR/4
  Short_BC/1 -> Vector Concatenate/5, OR/5
  Short_CA/1 -> OR/6, Vector Concatenate/6
  Constant36/1 -> Vector Concatenate/31
  Open_Bn/1 -> OR/11, Vector Concatenate/11
  Open_An/1 -> OR/10, Vector Concatenate/10
  Open_Ap/1 -> OR/7, Vector Concatenate/7
  Close_An/1 -> OR/16, Vector Concatenate/16
  Close_Ap/1 -> OR/13, Vector Concatenate/13
  Close_Cn/1 -> OR/18, Vector Concatenate/18
  Close_Bn/1 -> OR/17, Vector Concatenate/17
  Close_Cp/1 -> OR/15, Vector Concatenate/15
  Close_Bp/1 -> OR/14, Vector Concatenate/14
  Constant15/1 -> Vector Concatenate/24
  Constant14/1 -> Vector Concatenate/23
  Constant21/1 -> Vector Concatenate/20
  Constant20/1 -> Vector Concatenate/19
  Constant25/1 -> Vector Concatenate/26
  Constant24/1 -> Vector Concatenate/25
  Constant23/1 -> Vector Concatenate/22
  Constant22/1 -> Vector Concatenate/21
  Constant35/1 -> Vector Concatenate/30
  Constant34/1 -> Vector Concatenate/29
  Constant33/1 -> Vector Concatenate/28
  Constant32/1 -> Vector Concatenate/27
  Enable_Fault_UI/1 -> AND/3, Switch/2
  Vector Concatenate/1 -> Bit to Integer Converter/1
  Switch/1 -> Faults/1
  Bit to Integer Converter/1 -> Switch/1
  Constant1/1 -> Switch/3
  OR/1 -> AND/1
  AND/1 -> Terminator/1  "Fault_Present"
  Constant2/1 -> AND/2, Vector Concatenate/32

== system Copy_of_VTOLTiltrotor/Motor Control/Fault Trigering3 ==
  AND : Logic  Inputs=3  IconShape=distinctive  AllPortsSameDT=off  OutDataTypeStr=boolean
  Bit to Integer Converter : simulink/Logic and Bit Operations/Bit to Integer Converter  nbits=32  bitOrder=LSB first  signedOutputValues=Unsigned  outDtype=uint32  outDtypeSigned=Inherit via internal rule
  Close_An : Constant  Value=0  OutDataTypeStr=boolean  SampleTime=Ts_UI
  Close_Ap : Constant  Value=0  OutDataTypeStr=boolean  SampleTime=Ts_UI
  Close_Bn : Constant  Value=0  OutDataTypeStr=boolean  SampleTime=Ts_UI
  Close_Bp : Constant  Value=0  OutDataTypeStr=boolean  SampleTime=Ts_UI
  Close_Cn : Constant  Value=0  OutDataTypeStr=boolean  SampleTime=Ts_UI
  Close_Cp : Constant  Value=0  OutDataTypeStr=boolean  SampleTime=Ts_UI
  Constant1 : Constant  Value=0  OutDataTypeStr=uint32
  Constant{14..15,20..25,32..36} (13 alike) : Constant  Value=0  OutDataTypeStr=boolean  SampleTime=Ts_UI
  Constant2 : Constant  OutDataTypeStr=boolean  SampleTime=Ts_UI
  Enable_Fault_UI : Constant  OutDataTypeStr=boolean  SampleTime=Ts_UI
  OR : Logic  Operator=OR  Inputs=18  IconShape=distinctive  AllPortsSameDT=off  OutDataTypeStr=boolean
  Open_An : Constant  Value=0  OutDataTypeStr=boolean  SampleTime=Ts_UI
  Open_Ap : Constant  Value=0  OutDataTypeStr=boolean  SampleTime=Ts_UI
  Open_Bn : Constant  Value=0  OutDataTypeStr=boolean  SampleTime=Ts_UI
  Open_Bp : Constant  Value=0  OutDataTypeStr=boolean  SampleTime=Ts_UI
  Open_Cn : Constant  Value=0  OutDataTypeStr=boolean  SampleTime=Ts_UI
  Open_Cp : Constant  Value=0  OutDataTypeStr=boolean  SampleTime=Ts_UI
  Short_A : Constant  Value=0  OutDataTypeStr=boolean  SampleTime=Ts_UI
  Short_AB : Constant  Value=0  OutDataTypeStr=boolean  SampleTime=Ts_UI
  Short_B : Constant  Value=0  OutDataTypeStr=boolean  SampleTime=Ts_UI
  Short_BC : Constant  Value=0  OutDataTypeStr=boolean  SampleTime=Ts_UI
  Short_C : Constant  Value=0  OutDataTypeStr=boolean  SampleTime=Ts_UI
  Short_CA : Constant  Value=0  OutDataTypeStr=boolean  SampleTime=Ts_UI
  Switch : Switch  Criteria=u2 > Threshold  SaturateOnIntegerOverflow=off  InputSameDT=off
  Terminator : Terminator
  Vector Concatenate : Concatenate  NumInputs=32
  Faults : Outport
  wires:
  Open_Cn/1 -> OR/12, Vector Concatenate/12
  Open_Cp/1 -> OR/9, Vector Concatenate/9
  Short_A/1 -> OR/1, Vector Concatenate/1
  Open_Bp/1 -> OR/8, Vector Concatenate/8
  Short_B/1 -> Vector Concatenate/2, OR/2
  Short_C/1 -> Vector Concatenate/3, OR/3
  Short_AB/1 -> Vector Concatenate/4, OR/4
  Short_BC/1 -> Vector Concatenate/5, OR/5
  Short_CA/1 -> OR/6, Vector Concatenate/6
  Constant36/1 -> Vector Concatenate/31
  Open_Bn/1 -> OR/11, Vector Concatenate/11
  Open_An/1 -> OR/10, Vector Concatenate/10
  Open_Ap/1 -> OR/7, Vector Concatenate/7
  Close_An/1 -> OR/16, Vector Concatenate/16
  Close_Ap/1 -> OR/13, Vector Concatenate/13
  Close_Cn/1 -> OR/18, Vector Concatenate/18
  Close_Bn/1 -> OR/17, Vector Concatenate/17
  Close_Cp/1 -> OR/15, Vector Concatenate/15
  Close_Bp/1 -> OR/14, Vector Concatenate/14
  Constant15/1 -> Vector Concatenate/24
  Constant14/1 -> Vector Concatenate/23
  Constant21/1 -> Vector Concatenate/20
  Constant20/1 -> Vector Concatenate/19
  Constant25/1 -> Vector Concatenate/26
  Constant24/1 -> Vector Concatenate/25
  Constant23/1 -> Vector Concatenate/22
  Constant22/1 -> Vector Concatenate/21
  Constant35/1 -> Vector Concatenate/30
  Constant34/1 -> Vector Concatenate/29
  Constant33/1 -> Vector Concatenate/28
  Constant32/1 -> Vector Concatenate/27
  Enable_Fault_UI/1 -> AND/3, Switch/2
  Vector Concatenate/1 -> Bit to Integer Converter/1
  Switch/1 -> Faults/1
  Bit to Integer Converter/1 -> Switch/1
  Constant1/1 -> Switch/3
  OR/1 -> AND/1
  AND/1 -> Terminator/1  "Fault_Present"
  Constant2/1 -> AND/2, Vector Concatenate/32

== system Copy_of_VTOLTiltrotor/Motor Control/Motor Model Feedback ==
  Ia : Inport
  Ib : Inport  Port=2
  Ic : Inport  Port=3
  Motor_SPD_rads : Inport  Port=4
  Rate Transition{,1..3} (4 alike) : RateTransition  OutPortSampleTime=Ts_UI_fast
  Terminator{,1..3} (4 alike) : Terminator
  radsTOrpm : Gain  Gain=60/(2*pi)
  wires:
  Rate Transition1/1 -> Terminator/1  "Ia"
  Rate Transition3/1 -> Terminator2/1  "Ic"
  Rate Transition2/1 -> Terminator1/1  "Ib"
  Ib/1 -> Rate Transition2/1
  Ia/1 -> Rate Transition1/1
  Ic/1 -> Rate Transition3/1
  Motor_SPD_rads/1 -> Rate Transition/1
  radsTOrpm/1 -> Terminator3/1  "Motor Speed RPM"
  Rate Transition/1 -> radsTOrpm/1

== system Copy_of_VTOLTiltrotor/Motor Control/Motor Model Feedback1 ==
  Ia : Inport
  Ib : Inport  Port=2
  Ic : Inport  Port=3
  Motor_SPD_rads : Inport  Port=4
  Rate Transition{,1..3} (4 alike) : RateTransition  OutPortSampleTime=Ts_UI_fast
  Terminator{,1..3} (4 alike) : Terminator
  radsTOrpm : Gain  Gain=60/(2*pi)
  wires:
  Rate Transition1/1 -> Terminator/1  "Ia"
  Rate Transition3/1 -> Terminator2/1  "Ic"
  Rate Transition2/1 -> Terminator1/1  "Ib"
  Ib/1 -> Rate Transition2/1
  Ia/1 -> Rate Transition1/1
  Ic/1 -> Rate Transition3/1
  Motor_SPD_rads/1 -> Rate Transition/1
  radsTOrpm/1 -> Terminator3/1  "Motor Speed RPM"
  Rate Transition/1 -> radsTOrpm/1

== system Copy_of_VTOLTiltrotor/Motor Control/Motor Model Feedback2 ==
  Ia : Inport
  Ib : Inport  Port=2
  Ic : Inport  Port=3
  Motor_SPD_rads : Inport  Port=4
  Rate Transition{,1..3} (4 alike) : RateTransition  OutPortSampleTime=Ts_UI_fast
  Terminator{,1..3} (4 alike) : Terminator
  radsTOrpm : Gain  Gain=60/(2*pi)
  wires:
  Rate Transition1/1 -> Terminator/1  "Ia"
  Rate Transition3/1 -> Terminator2/1  "Ic"
  Rate Transition2/1 -> Terminator1/1  "Ib"
  Ib/1 -> Rate Transition2/1
  Ia/1 -> Rate Transition1/1
  Ic/1 -> Rate Transition3/1
  Motor_SPD_rads/1 -> Rate Transition/1
  radsTOrpm/1 -> Terminator3/1  "Motor Speed RPM"
  Rate Transition/1 -> radsTOrpm/1

== system Copy_of_VTOLTiltrotor/Motor Control/Motor Model Feedback3 ==
  Ia : Inport
  Ib : Inport  Port=2
  Ic : Inport  Port=3
  Motor_SPD_rads : Inport  Port=4
  Rate Transition{,1..3} (4 alike) : RateTransition  OutPortSampleTime=Ts_UI_fast
  Terminator{,1..3} (4 alike) : Terminator
  radsTOrpm : Gain  Gain=60/(2*pi)
  wires:
  Rate Transition1/1 -> Terminator/1  "Ia"
  Rate Transition3/1 -> Terminator2/1  "Ic"
  Rate Transition2/1 -> Terminator1/1  "Ib"
  Ib/1 -> Rate Transition2/1
  Ia/1 -> Rate Transition1/1
  Ic/1 -> Rate Transition3/1
  Motor_SPD_rads/1 -> Rate Transition/1
  radsTOrpm/1 -> Terminator3/1  "Motor Speed RPM"
  Rate Transition/1 -> radsTOrpm/1

== system Copy_of_VTOLTiltrotor/Motor Control/Three-Phase PMSM Drive ==
  V_dc : Inport
  Fault : Inport  Port=2
  LdTrq/Spd : Inport  Port=3
  Simu_config : Inport  Port=4
  PMSM and average inverter : Subsystem  VariantControl=str2num(get_param(['VTOLTiltrotor/Motor Control/SimulationVariant'], 'Value'))==1
  PMSM and inverter with switching dynamics : Subsystem  VariantControl=str2num(get_param(['VTOLTiltrotor/Motor Control/SimulationVariant'], 'Value'))>1
  Ia : Outport
  Ib : Outport  Port=2
  Ic : Outport  Port=3
  Motor_Spd : Outport  Port=4
  Motor_Angle : Outport  Port=5
  QAE_Pos_C : Outport  Port=6

== system Copy_of_VTOLTiltrotor/Motor Control/Three-Phase PMSM Drive1 ==
  V_dc : Inport
  Fault : Inport  Port=2
  LdTrq/Spd : Inport  Port=3
  Simu_config : Inport  Port=4
  PMSM and average inverter : Subsystem  VariantControl=str2num(get_param(['VTOLTiltrotor/Motor Control/SimulationVariant'], 'Value'))==1
  Ia : Outport
  Ib : Outport  Port=2
  Ic : Outport  Port=3
  Motor_Spd : Outport  Port=4
  Motor_Angle : Outport  Port=5
  QAE_Pos_C : Outport  Port=6

== system Copy_of_VTOLTiltrotor/Motor Control/Three-Phase PMSM Drive2 ==
  V_dc : Inport
  Fault : Inport  Port=2
  LdTrq/Spd : Inport  Port=3
  Simu_config : Inport  Port=4
  PMSM and average inverter : Subsystem  VariantControl=str2num(get_param(['VTOLTiltrotor/Motor Control/SimulationVariant'], 'Value'))==1
  Ia : Outport
  Ib : Outport  Port=2
  Ic : Outport  Port=3
  Motor_Spd : Outport  Port=4
  Motor_Angle : Outport  Port=5
  QAE_Pos_C : Outport  Port=6

== system Copy_of_VTOLTiltrotor/Motor Control/Three-Phase PMSM Drive3 ==
  V_dc : Inport
  Fault : Inport  Port=2
  LdTrq/Spd : Inport  Port=3
  Simu_config : Inport  Port=4
  PMSM and average inverter : Subsystem  VariantControl=str2num(get_param(['VTOLTiltrotor/Motor Control/SimulationVariant'], 'Value'))==1
  Ia : Outport
  Ib : Outport  Port=2
  Ic : Outport  Port=3
  Motor_Spd : Outport  Port=4
  Motor_Angle : Outport  Port=5
  QAE_Pos_C : Outport  Port=6

== system Copy_of_VTOLTiltrotor/Motor Control/User Interface ==
  note: Fault Present
  note: Hardware-in-the-Loop
      | Motor & Inverter
      | Real-Time Simulation
  note: Motor Currents [A]
  note: Model Response
  note: Kp
  note: UI Speed Command enabled
  note: Tx: Message to Controller
  note: Speed Controller PI Gain Tuning
  note: Ki
  note: Rx: Message From Controller
  note: Open A-
  note: Open C-
  note: Short AB
  note: Short B
  note: Short CA
  note: Open A+
  note: Short BC
  note: Open B-
  note: Open B+
  note: Open C+
  note: Short A
  note: Short C
  note: Inverter Faults
  note: Motor Speed [rpm]
  note: Time [s]
  note: Time [s]
  note: Time [s]
  note: Motor Speed [rpm]
  note: Encoder Count [steps]
  note: (only for switching inverter)
  note: (only short A with included bitstream)
  Dashboard Scope1 : DashboardScope  ShowInitialText=off  TimeSpan=0.10000000000000001  Ymin=-50  Ymax=50  ScaleAtStop=off  UpdateMode=Scroll
  Dashboard Scope2 : DashboardScope  ShowInitialText=off  TimeSpan=1  Ymin=0  Ymax=1e5  ScaleAtStop=off
  Dashboard Scope3 : DashboardScope  ShowInitialText=off  TimeSpan=10  Ymin=0  Ymax=3000  ScaleAtStop=off
  Edit : EditField  LabelPosition=Hide  ShowInitialText=on  Alignment=Center
  Edit1 : EditField  LabelPosition=Hide  ShowInitialText=on  Alignment=Center
  Faults Enabled : SliderSwitchBlock  LabelPosition=Hide
      settings: Values={{'Faults UI OFF', 'Faults UI ON'}, [0 1]}
  Gauge : CircularGaugeBlock  LabelPosition=Hide  ScaleMin=-3000  ScaleMax=3000
  Lamp : LampBlock  LabelPosition=Hide
  Lamp1 : LampBlock  LabelPosition=Hide
  Lamp2 : LampBlock  LabelPosition=Hide
  Open An : ToggleSwitchBlock  LabelPosition=Hide
      settings: Values={{'Off', 'On'}, [0 1]}
  Open Ap : ToggleSwitchBlock  LabelPosition=Hide
      settings: Values={{'Off', 'On'}, [0 1]}
  Open Bn : ToggleSwitchBlock  LabelPosition=Hide
      settings: Values={{'Off', 'On'}, [0 1]}
  Open Bp : ToggleSwitchBlock  LabelPosition=Hide
      settings: Values={{'Off', 'On'}, [0 1]}
  Open Cn : ToggleSwitchBlock  LabelPosition=Hide
      settings: Values={{'Off', 'On'}, [0 1]}
  Open Cp : ToggleSwitchBlock  LabelPosition=Hide
      settings: Values={{'Off', 'On'}, [0 1]}
  Short A : ToggleSwitchBlock  LabelPosition=Hide
      settings: Values={{'Off', 'On'}, [0 1]}
  Short AB : ToggleSwitchBlock  LabelPosition=Hide
      settings: Values={{'Off', 'On'}, [0 1]}
  Short B : ToggleSwitchBlock  LabelPosition=Hide
      settings: Values={{'Off', 'On'}, [0 1]}
  Short BC : ToggleSwitchBlock  LabelPosition=Hide
      settings: Values={{'Off', 'On'}, [0 1]}
  Short C : ToggleSwitchBlock  LabelPosition=Hide
      settings: Values={{'Off', 'On'}, [0 1]}
  Short CA : ToggleSwitchBlock  LabelPosition=Hide
      settings: Values={{'Off', 'On'}, [0 1]}
  Slider : SliderBlock  LabelPosition=Hide  ScaleMin=1e-5  ScaleMax=10  ScaleType=Log
  Slider Switch : SliderSwitchBlock  LabelPosition=Hide
      settings: Values={{'Sinus Open Loop', 'FOC Closed Loop'}, [0 1]}
  Slider Switch1 : SliderSwitchBlock  LabelPosition=Hide
      settings: Values={{'PWM OFF', 'PWM ON'}, [0 1]}
  Slider Switch2 : SliderSwitchBlock  LabelPosition=Hide
      settings: Values={{'Default Values', 'Live Tuning'}, [1 0]}
  Slider1 : SliderBlock  LabelPosition=Hide  ScaleMin=1e-5  ScaleMax=10  ScaleType=Log

== system Copy_of_VTOLTiltrotor/Visualization/No Visualization ==
  UAVState : Inport
  Terminator : Terminator
  wires:
  UAVState/1 -> Terminator/1
